simulink library "helperTrafficLightControllerLib"  (R2023b)
settings: Solver=VariableStepAuto  StartTime=0.0  StopTime=10.0  RelTol=1e-3
libraries: sim3dlib x2
settings Model: Creator=The MathWorks, Inc.  LastModifiedBy=The MathWorks, Inc.
settings SolverCC: AlgebraicLoopSolver=TrustRegion
settings DebuggingCC: UnconnectedInputMsg=warning  UnconnectedOutputMsg=warning  UnconnectedLineMsg=warning  SubsystemReferenceDiagnosticForUnitTest=warning
settings ModelReferenceCC: EnableRefExpFcnMdlSchedulingChecks=on

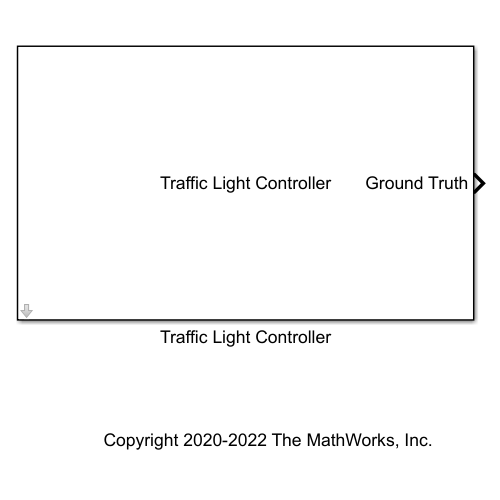
[thumbnail: Simulink's stored preview of the top-level diagram]
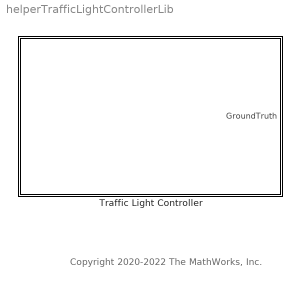
== system helperTrafficLightControllerLib ==
  note: Copyright 2020-2022 The MathWorks, Inc.
  Traffic Light Controller : Subsystem  Priority=-1  mask(Traffic Light Controller){helperTrafficLightCheck=0, customScene=0, modeType=Timer-based, vehTagList={'Scene Origin';'SimulinkVehicle1'}, MsgSize=[1 62], vehTag=SimulinkVehicle1, trafficLightID=1, greenTime=10, yellowTime=3, redClearanceTime=0, aMode=3, Ts=-1}
      mask prompts: modeType "shared_sim3dblks:sim3dblkHelperTrafficLightController:blkPrm_modeType"; MsgSize "shared_sim3dblks:sim3dblkMessageGET:blkPrm_MsgSize"; vehTag "shared_sim3dblks:sim3dblkHelperTrafficLightController:blkPrm_vehTag"; trafficLightID "shared_sim3dblks:sim3dblkHelperTrafficLightController:blkPrm_trafficLightID"; greenTime "shared_sim3dblks:sim3dblkHelperTrafficLightController:blkPrm_greenTime"; yellowTime "shared_sim3dblks:sim3dblkHelperTrafficLightController:blkPrm_yellowTime"; redClearanceTime "shared_sim3dblks:sim3dblkHelperTrafficLightController:blkPrm_redTime"; Ts "shared_sim3dblks:sim3dblkMessageGET:blkPrm_Ts"
      mask help: shared_sim3dblks:sim3dblkHelperTrafficLightController:blkDesc
      mask init:
      | sim3dblkssharedicon('sim3dblkshelpertrafficlightcontroller',gcb,'Initialization');
      mask Help: helpview(fullfile(docroot,'toolbox','driving','helptargets.map'),'HighwayLaneFollowingExample')
      mask TypeOptions modeType: Timer-based | Event-based | State-based
      mask Callback modeType: sim3dblkssharedicon('sim3dblkshelpertrafficlightcontroller', gcb, 'UpdateFieldsMode');
      mask Callback vehTagList: sim3dblkssharedicon('sim3dblkshelpertrafficlightcontroller', gcb, 'InitVehTagList');
      mask TypeOptions MsgSize: Simulation 3D Message Get1/MsgSize
      mask TypeOptions vehTag: - Select Vehicle - | SimulinkVehicle1 | EgoVehicle | LeadVehicle
      mask TypeOptions Ts: Simulation 3D Message Get1/Ts | Simulation 3D Message Set1/Ts
      mask DialogControl DescGroupVar Prompt: Traffic Light Controller
      mask DialogControl DescTextVar Prompt: shared_sim3dblks:sim3dblkHelperTrafficLightController:blkDesc
      mask DialogControl Container Prompt: Parameter
      mask DialogControl modeType Prompt: Control mode:
      mask DialogControl MsgSize Prompt: Message size, MsgSize []:
      mask DialogControl vehTag Prompt: Select Vehicle:
      mask DialogControl trafficLightID Prompt: Traffic light ID:
      mask DialogControl greenTime Prompt: Green time (sec):
      mask DialogControl yellowTime Prompt: Yellow time (sec):
      mask DialogControl redClearanceTime Prompt: Red clearance time (sec):
      mask DialogControl Ts Prompt: Sample time:
      mask Display:
      | disp(['Traffic Light Controller']);
      | i=1;
      | j=1;
      | mode= get_param(gcb,'modeType');
      | if strcmp(mode,'State-based')
      |     port_label('output',j,'Ground Truth');
      |     port_label('input',i,'Traffic Light ID');
      |     port_label('input',i+1,'State');
      | elseif strcmp(mode,'Event-based')
      |     port_label('input',i,'Distance');
      |     port_label('input',i+1,'State');
      |     port_label('output',j,'Ground Truth');
      |     port_label('output',j+1,'Upcoming Traffic Light ID');
      | elseif strcmp(mode,'Timer-based')
      |     port_label('output',j,'Ground Truth');
      | end

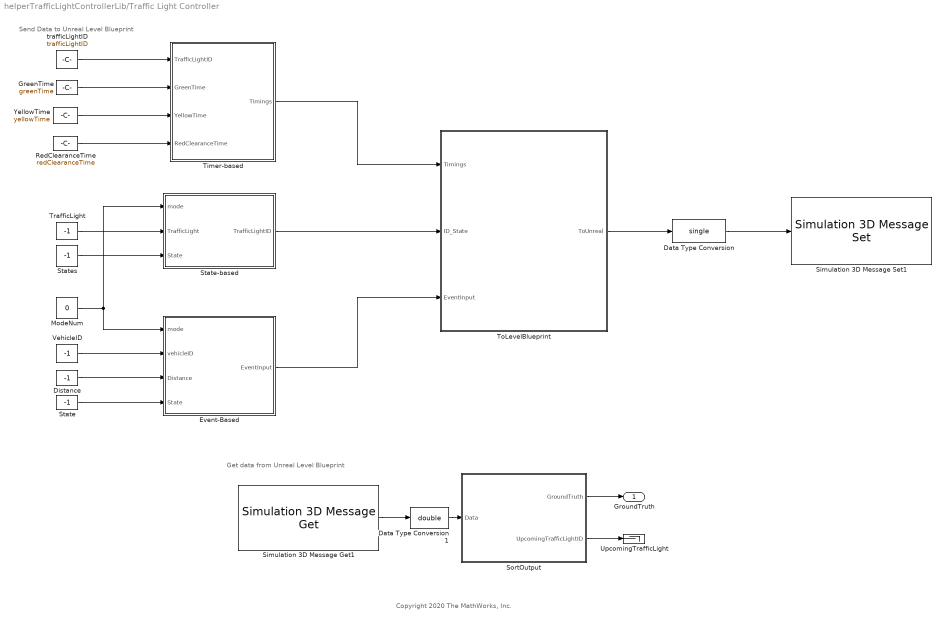
== system helperTrafficLightControllerLib/Traffic Light Controller ==
  note: Get data from Unreal Level Blueprint
  note: Send Data to Unreal Level Blueprint
  note: Copyright 2020 The MathWorks, Inc.
  Data Type Conversion : DataTypeConversion  OutDataTypeStr=single  SaturateOnIntegerOverflow=off  RndMeth=Floor
  Data Type Conversion1 : DataTypeConversion  OutDataTypeStr=double  SaturateOnIntegerOverflow=off  RndMeth=Floor
  Distance : Constant  Value=-1
  Event-Based : MATLAB Function  TreatAsAtomicUnit=on
  GreenTime : Constant  Value=greenTime
  ModeNum : Constant  Value=0
  RedClearanceTime : Constant  Value=redClearanceTime
  Simulation 3D Message Get1 : sim3dlib/Simulation 3D Message Get  Priority=-1  SigName=getTrafficLights  DataType=single  MsgSize=MsgSize  Ts=Ts  aMode=aMode
  Simulation 3D Message Set1 : sim3dlib/Simulation 3D Message Set  Priority=-1  SigName=setTrafficLights  Ts=Ts  aMode=aMode
  SortOutput : MATLAB Function  TreatAsAtomicUnit=on
  State : Constant  Value=-1
  State-based : MATLAB Function  TreatAsAtomicUnit=on
  States : Constant  Value=-1
  Timer-based : MATLAB Function  TreatAsAtomicUnit=on
  ToLevelBlueprint : MATLAB Function  TreatAsAtomicUnit=on
  TrafficLight : Constant  Value=-1
  UpcomingTrafficLight : Terminator
  VehicleID : Constant  Value=-1
  YellowTime : Constant  Value=yellowTime
  trafficLightID : Constant  Value=trafficLightID
  GroundTruth : Outport
  wires:
  ToLevelBlueprint/1(ToUnreal) -> Data Type Conversion/1
  Data Type Conversion/1 -> Simulation 3D Message Set1/1
  Simulation 3D Message Get1/1 -> Data Type Conversion1/1
  SortOutput/1(GroundTruth) -> GroundTruth/1
  States/1 -> State-based/3(State)
  SortOutput/2(UpcomingTrafficLightID) -> UpcomingTrafficLight/1
  trafficLightID/1 -> Timer-based/1(TrafficLightID)
  GreenTime/1 -> Timer-based/2(GreenTime)
  YellowTime/1 -> Timer-based/3(YellowTime)
  RedClearanceTime/1 -> Timer-based/4(RedClearanceTime)
  Data Type Conversion1/1 -> SortOutput/1(Data)
  TrafficLight/1 -> State-based/2(TrafficLight)
  State-based/1(TrafficLightID) -> ToLevelBlueprint/2(ID_State)
  VehicleID/1 -> Event-Based/2(vehicleID)
  Distance/1 -> Event-Based/3(Distance)
  State/1 -> Event-Based/4(State)
  Event-Based/1(EventInput) -> ToLevelBlueprint/3(EventInput)
  Timer-based/1(Timings) -> ToLevelBlueprint/1(Timings)
  ModeNum/1 -> Event-Based/1(mode), State-based/1(mode)

== matlab function helperTrafficLightControllerLib/Traffic Light Controller/Event-Based ==
  data: mode input; EventInput output; vehicleID input; Distance input size=[1 1] [1..100]; State input size=[1 1] [0..2]
function EventInput = Event_Based(mode, vehicleID, Distance, State)
%   Event_Based converts vehicleID, Distance and State into a row vector

%   Copyright 2020 The MathWorks, Inc.

coder.extrinsic('message')
if mode==1
    if ~(Distance>=1 && Distance<=100)
        pause(0.5);
        error(message('shared_sim3dblks:sim3dblkHelperTrafficLightController:invalidDistance'));
    elseif ~(State>=0&&State<=2)
        pause(0.5);
        error(message('shared_sim3dblks:sim3dblkHelperTrafficLightController:invalidState'));
    elseif ~(mod(State,1)==0)
        pause(0.5);
        error(message('shared_sim3dblks:sim3dblkHelperTrafficLightController:invalidState'));
    end
end
EventInput=[vehicleID Distance State];

== matlab function helperTrafficLightControllerLib/Traffic Light Controller/SortOutput ==
  data: Data input; GroundTruth output; UpcomingTrafficLightID output
function [GroundTruth,UpcomingTrafficLightID] = LevelBlueprint(Data)
%   LevelBlueprint seperates incoming Data into GroundTruth and
%   UpcomingTrafficLightID

%   Copyright 2020 The MathWorks, Inc.

GroundTruth=reshape(Data(3:end),2,[])';
GroundTruth=sortrows(GroundTruth,1);
UpcomingTrafficLightID=Data(2);
end

== matlab function helperTrafficLightControllerLib/Traffic Light Controller/State-based ==
  data: mode input; TrafficLight input; TrafficLightID output; State input [0..2]
function TrafficLightID = StateBased(mode,TrafficLight,State)
%   StateBased converts TrafficLight and State to a row vector

%   Copyright 2020 The MathWorks, Inc.

coder.extrinsic('message')


if mode==2
    if ~(all(TrafficLight>=1) && all(TrafficLight<=200)) || ~all(mod(TrafficLight,1)==0)
        pause(0.5);
        error(message('shared_sim3dblks:sim3dblkHelperTrafficLightController:invalidTrafficLightID'));
    end
    if ~(size(State,2)==1)
        pause(0.5);
        error(message('shared_sim3dblks:sim3dblkHelperTrafficLightController:invalidStatesSize'));
    end
    if ~(size(TrafficLight,2)==1)
        pause(0.5);
        error(message('shared_sim3dblks:sim3dblkHelperTrafficLightController:invalidTrafficLightIDSize'));
    end
    if ~(all(State>=0) && all(State<=2)) || ~all(mod(State,1)==0)
        pause(0.5);
        error(message('shared_sim3dblks:sim3dblkHelperTrafficLightController:invalidState'));
    end

    if ~(length(TrafficLight)==length(State))
        pause(0.5);
        error(message('shared_sim3dblks:sim3dblkHelperTrafficLightController:invalidIDStateSize'));
    end
end
TrafficLight=reshape(TrafficLight,1,length(TrafficLight));
State=reshape(State,1,length(State));
TrafficLightID=[TrafficLight State];

== matlab function helperTrafficLightControllerLib/Traffic Light Controller/Timer-based ==
  data: TrafficLightID input; Timings output; GreenTime input; YellowTime input; RedClearanceTime input
function Timings = TimerBased(TrafficLightID,GreenTime,YellowTime,RedClearanceTime)
%   TimerBased converts TrafficLightID, GreenTime, YellowTime and
%   RedClearanceTime to a row vector.

%   Copyright 2020 The MathWorks, Inc.

sort_Timings = [TrafficLightID GreenTime YellowTime RedClearanceTime];
Timings=reshape(sort_Timings',1,[]);

== matlab function helperTrafficLightControllerLib/Traffic Light Controller/ToLevelBlueprint ==
  data: Timings input; ID_State input; EventInput input; ToUnreal output
function ToUnreal = inputToUnreal(Timings, ID_State, EventInput)
%   inputToUnreal converts Timings, ID_State, EventInput to a single row
%   vector. Also it includes the matrix(Timings) length and stateLength in
%   the row vector

%   Copyright 2020-2022 The MathWorks, Inc.

matrixLength=length(Timings)/4;
statesLength=length(ID_State)/2;
actualData = [EventInput statesLength matrixLength ID_State Timings];
zerosRequired = 76-length(actualData);
ToUnreal = [actualData zeros(1,zerosRequired)];
